simulink model "heli_trim"  (Simulink 7.7)
settings: Solver=FixedStepDiscrete  StartTime=0.0  StopTime=in_N  FixedStep=1  RelTol=1e-3
PostLoadFcn:
  | if exist('helicopter_trim.mat', 'file')
  |     load helicopter_trim.mat;
  | end
undefined symbols (not defined in the file or in its folder): alpha_IERA_IELA_IELA, in_CMD_ini, in_omega_MR, in_omega_TR, in_outside_air_temp, in_pressure_altitude, R_IERA_RA_RA
libraries: UAVdesign_net x2, simulink x2
settings Model: Creator=Emanuel  LastModifiedBy=Emanuel
settings DataIOCC: LimitDataPoints=off  SaveOutput=off  SignalLogging=off
settings OptimizationCC: SimCompilerOptimization=On
settings DebuggingCC: StrictBusMsg=Warning
settings HardwareCC: ProdIntDivRoundTo=Zero  ProdEndianess=LittleEndian  ProdHWDeviceType=Generic->32-bit x86 compatible
settings SFSimCC: SimParseCustomCode=off

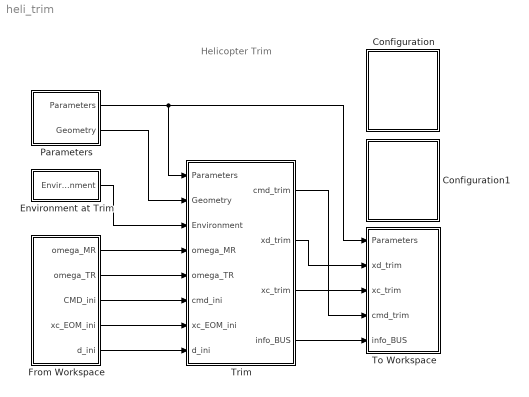
== system heli_trim ==
  note: Helicopter Trim
  Configuration : Subsystem
      settings: OpenFcn=gui_HelicopterTrim;
      mask Display: disp('Double-click\nto configure\nthe\nsimulation')
  Configuration1 : Subsystem
      settings: OpenFcn=graphs_Helicopter_trim;
      mask Display: disp('Double-click\nto display\nthe\ngraphs')
  Environment at Trim : Subsystem
  From Workspace : Subsystem
  Parameters : Subsystem
      mask init:
      | set_param(gcb, 'LinkStatus', 'none');
      settings: OpenFcn=gui_HelicopterParameters( 'Block', [get_param(gcb, 'Parent') '/' get_param(gcb, 'Name')]);
      mask Display:
      | port_label('output', 1, 'Parameters')
      | port_label('output', 2, 'Geometry')
  To Workspace : Subsystem
  Trim : Subsystem  TreatAsAtomicUnit=on
  wires:
  Parameters/2(Geometry) -> Trim/2(Geometry)
  Parameters/1(Parameters) -> Trim/1(Parameters), To Workspace/1(Parameters)
  Trim/2(xd_trim) -> To Workspace/2(xd_trim)
  From Workspace/3(CMD_ini) -> Trim/6(cmd_ini)
  From Workspace/4(xc_EOM_ini) -> Trim/7(xc_EOM_ini)
  From Workspace/5(d_ini) -> Trim/8(d_ini)
  Trim/1(cmd_trim) -> To Workspace/4(cmd_trim)
  Environment at Trim/1(Environment) -> Trim/3(Environment)
  From Workspace/2(omega_TR) -> Trim/5(omega_TR)
  From Workspace/1(omega_MR) -> Trim/4(omega_MR)
  Trim/4(info_BUS) -> To Workspace/5(info_BUS)
  Trim/3(xc_trim) -> To Workspace/3(xc_trim)

== system heli_trim/Configuration ==

== system heli_trim/Configuration1 ==

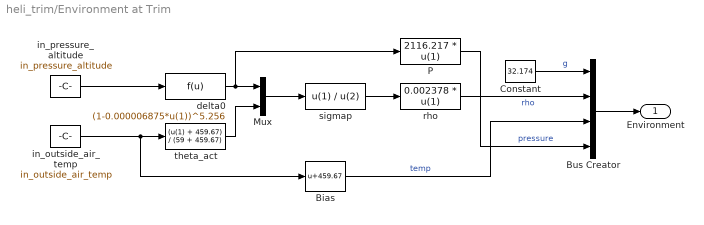
== system heli_trim/Environment at Trim ==
  Bias : Bias  Bias=459.67
  Bus Creator : BusCreator  OutDataTypeStr=Bus: Environment  NonVirtualBus=on
  Constant : Constant  Value=32.174
  Mux : Mux  Inputs=2
  P : Fcn  Expr=2116.217 * u(1)
  delta0 : Fcn  Expr=(1-0.000006875*u(1))^5.256
  in_outside_air_temp : Constant  Value=in_outside_air_temp
  in_pressure_altitude : Constant  Value=in_pressure_altitude
  rho : Fcn  Expr=0.002378 * u(1)
  sigmap : Fcn  Expr=u(1) / u(2)
  theta_act : Fcn  Expr=(u(1) + 459.67) / (59 + 459.67)
  Environment : Outport  OutDataTypeStr=Bus: Environment
  wires:
  sigmap/1 -> rho/1
  theta_act/1 -> Mux/2
  Mux/1 -> sigmap/1
  in_outside_air_temp/1 -> Bias/1, theta_act/1
  delta0/1 -> P/1, Mux/1
  in_pressure_altitude/1 -> delta0/1
  Bus Creator/1 -> Environment/1
  Constant/1 -> Bus Creator/1  "g"
  rho/1 -> Bus Creator/2  "rho"
  Bias/1 -> Bus Creator/3  "temp"
  P/1 -> Bus Creator/4  "pressure"

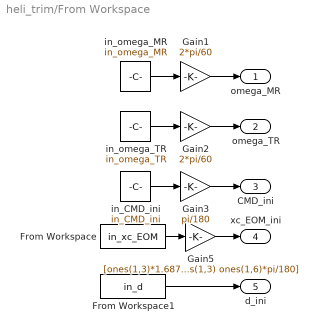
== system heli_trim/From Workspace ==
  From Workspace : FromWorkspace  VariableName=in_xc_EOM  SampleTime=1
  From Workspace1 : FromWorkspace  VariableName=in_d  SampleTime=1
  Gain1 : Gain  Gain=2*pi/60
  Gain2 : Gain  Gain=2*pi/60
  Gain3 : Gain  Gain=pi/180
  Gain5 : Gain  Gain=[ones(1,3)*1.68780986 ones(1,3) ones(1,6)*pi/180]
  in_CMD_ini : Constant  Value=in_CMD_ini
  in_omega_MR : Constant  Value=in_omega_MR
  in_omega_TR : Constant  Value=in_omega_TR
  omega_MR : Outport
  omega_TR : Outport  Port=2
  CMD_ini : Outport  Port=3
  xc_EOM_ini : Outport  Port=4
  d_ini : Outport  Port=5
  wires:
  in_omega_MR/1 -> Gain1/1
  in_omega_TR/1 -> Gain2/1
  in_CMD_ini/1 -> Gain3/1
  From Workspace/1 -> Gain5/1
  Gain1/1 -> omega_MR/1
  Gain2/1 -> omega_TR/1
  Gain3/1 -> CMD_ini/1
  Gain5/1 -> xc_EOM_ini/1
  From Workspace1/1 -> d_ini/1

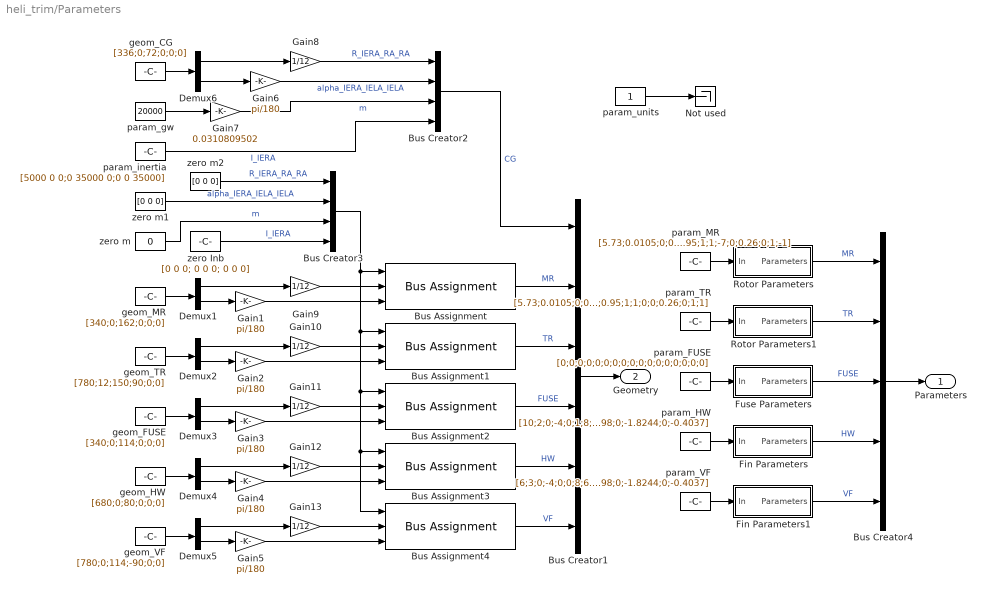
== system heli_trim/Parameters ==
  Bus Assignment{,1..4} (5 alike) : BusAssignment  AssignedSignals=R_IERA_RA_RA,alpha_IERA_IELA_IELA
  Bus Creator1 : BusCreator  Inputs=6
  Bus Creator2 : BusCreator  OutDataTypeStr=Bus: GeometryParameters
  Bus Creator3 : BusCreator  OutDataTypeStr=Bus: GeometryParameters
  Bus Creator4 : BusCreator  Inputs=5
  Demux{1..6} (6 alike) : Demux  Outputs=2
  Fin Parameters : Subsystem
  Fin Parameters1 : Subsystem
  Fuse Parameters : Subsystem
  Gain{1..6} (6 alike) : Gain  Gain=pi/180
  Gain{8..13} (6 alike) : Gain  Gain=1/12
  Gain7 : Gain  Gain=0.0310809502
  Not used : Terminator
  Rotor Parameters : Subsystem
  Rotor Parameters1 : Subsystem
  geom_CG : Constant  Value=[336;0;72;0;0;0]
  geom_FUSE : Constant  Value=[340;0;114;0;0;0]
  geom_HW : Constant  Value=[680;0;80;0;0;0]
  geom_MR : Constant  Value=[340;0;162;0;0;0]
  geom_TR : Constant  Value=[780;12;150;90;0;0]
  geom_VF : Constant  Value=[780;0;114;-90;0;0]
  param_FUSE : Constant  Value=[0;0;0;0;0;0;0;0;0;0;0;0;0;0;0;0;0]
  param_HW : Constant  Value=[10;2;0;-4;0;1;8;6.13;0.9682;1.8898;0;-1.8244;0;-0.4037]
  param_MR : Constant  Value=[5.73;0.0105;0;0.01325;0;-15;0;0;7;30;2.5;0.95;1;1;-7;0;0.26;0;1;-1]
  param_TR : Constant  Value=[5.73;0.0105;0;0.01325;0;-45;0;0;4;6.5;1.25;0.95;1;1;0;0;0.26;0;1;1]
  param_VF : Constant  Value=[6;3;0;-4;0;0;8;6.1311;0.9682;1.8898;0;-1.8244;0;-0.4037]
  param_gw : Constant  Value=20000
  param_inertia : Constant  Value=[5000 0 0;0 35000 0;0 0 35000]
  param_units : Constant
  zero Inb : Constant  Value=[0 0 0; 0 0 0; 0 0 0]
  zero m : Constant  Value=0
  zero m1 : Constant  Value=[0 0 0]
  zero m2 : Constant  Value=[0 0 0]
  Parameters : Outport
  Geometry : Outport  Port=2
  wires:
  Bus Creator2/1 -> Bus Creator1/1  "CG"
  Bus Assignment1/1 -> Bus Creator1/3  "TR"
  Bus Assignment2/1 -> Bus Creator1/4  "FUSE"
  Bus Assignment3/1 -> Bus Creator1/5  "HW"
  Bus Assignment4/1 -> Bus Creator1/6  "VF"
  Bus Creator1/1 -> Geometry/1
  Demux6/1 -> Gain8/1
  Demux6/2 -> Gain6/1
  param_gw/1 -> Gain7/1
  param_inertia/1 -> Bus Creator2/4  "I_IERA"
  Bus Assignment/1 -> Bus Creator1/2  "MR"
  Demux1/1 -> Gain9/1
  Demux1/2 -> Gain1/1
  geom_MR/1 -> Demux1/1
  Demux2/1 -> Gain10/1
  Demux2/2 -> Gain2/1
  geom_TR/1 -> Demux2/1
  Demux3/1 -> Gain11/1
  Demux3/2 -> Gain3/1
  geom_FUSE/1 -> Demux3/1
  Demux4/1 -> Gain12/1
  Demux4/2 -> Gain4/1
  geom_HW/1 -> Demux4/1
  Demux5/1 -> Gain13/1
  Demux5/2 -> Gain5/1
  geom_VF/1 -> Demux5/1
  geom_CG/1 -> Demux6/1
  Bus Creator3/1 -> Bus Assignment/1, Bus Assignment1/1, Bus Assignment2/1, Bus Assignment4/1, Bus Assignment3/1
  zero m/1 -> Bus Creator3/3  "m"
  zero m1/1 -> Bus Creator3/2  "alpha_IERA_IELA_IELA"
  zero Inb/1 -> Bus Creator3/4  "I_IERA"
  zero m2/1 -> Bus Creator3/1  "R_IERA_RA_RA"
  Bus Creator4/1 -> Parameters/1
  Rotor Parameters/1(Parameters) -> Bus Creator4/1  "MR"
  param_MR/1 -> Rotor Parameters/1(In)
  Rotor Parameters1/1(Parameters) -> Bus Creator4/2  "TR"
  param_TR/1 -> Rotor Parameters1/1(In)
  param_FUSE/1 -> Fuse Parameters/1(In)
  Fuse Parameters/1(Parameters) -> Bus Creator4/3  "FUSE"
  param_VF/1 -> Fin Parameters1/1(In)
  Fin Parameters1/1(Parameters) -> Bus Creator4/5  "VF"
  Fin Parameters/1(Parameters) -> Bus Creator4/4  "HW"
  param_HW/1 -> Fin Parameters/1(In)
  Gain1/1 -> Bus Assignment/3
  Gain2/1 -> Bus Assignment1/3
  Gain3/1 -> Bus Assignment2/3
  Gain4/1 -> Bus Assignment3/3
  Gain5/1 -> Bus Assignment4/3
  Gain6/1 -> Bus Creator2/2  "alpha_IERA_IELA_IELA"
  Gain7/1 -> Bus Creator2/3  "m"
  Gain8/1 -> Bus Creator2/1  "R_IERA_RA_RA"
  Gain9/1 -> Bus Assignment/2
  Gain10/1 -> Bus Assignment1/2
  Gain11/1 -> Bus Assignment2/2
  Gain12/1 -> Bus Assignment3/2
  Gain13/1 -> Bus Assignment4/2
  param_units/1 -> Not used/1

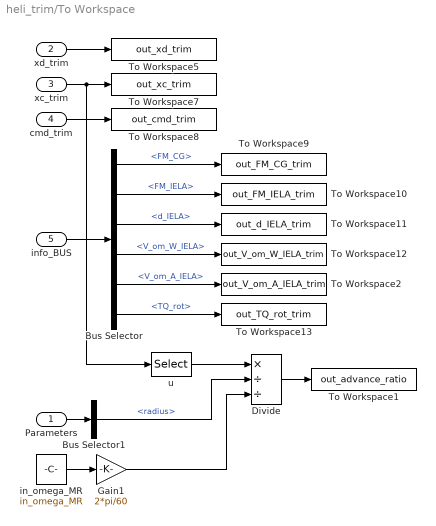
== system heli_trim/To Workspace ==
  Parameters : Inport
  xd_trim : Inport  Port=2
  xc_trim : Inport  Port=3
  cmd_trim : Inport  Port=4
  info_BUS : Inport  Port=5
  Bus Selector : BusSelector  OutputSignals=FM_CG,FM_IELA,d_IELA,V_om_W_IELA,V_om_A_IELA,TQ_rot
  Bus Selector1 : BusSelector  OutputSignals=MR.radius
  Divide : Product  Inputs=*//
  Gain1 : Gain  Gain=2*pi/60
  To Workspace1 : ToWorkspace  VariableName=out_advance_ratio  SampleTime=-1  SaveFormat=Array
  To Workspace10 : ToWorkspace  VariableName=out_FM_IELA_trim  SampleTime=-1  SaveFormat=Array
  To Workspace11 : ToWorkspace  VariableName=out_d_IELA_trim  SampleTime=-1  SaveFormat=Array
  To Workspace12 : ToWorkspace  VariableName=out_V_om_W_IELA_trim  SampleTime=-1  SaveFormat=Array
  To Workspace13 : ToWorkspace  VariableName=out_TQ_rot_trim  SampleTime=-1  SaveFormat=Array
  To Workspace2 : ToWorkspace  VariableName=out_V_om_A_IELA_trim  SampleTime=-1  SaveFormat=Array
  To Workspace5 : ToWorkspace  VariableName=out_xd_trim  SampleTime=-1  SaveFormat=Array
  To Workspace7 : ToWorkspace  VariableName=out_xc_trim  SampleTime=-1  SaveFormat=Array
  To Workspace8 : ToWorkspace  VariableName=out_cmd_trim  SampleTime=-1  SaveFormat=Array
  To Workspace9 : ToWorkspace  VariableName=out_FM_CG_trim  SampleTime=-1  SaveFormat=Array
  in_omega_MR : Constant  Value=in_omega_MR
  u : Selector  InputPortWidth=26  IndexOptions=Index vector (dialog)  Indices=[9]  OutputSizes=1
  wires:
  xd_trim/1 -> To Workspace5/1
  xc_trim/1 -> To Workspace7/1, u/1
  cmd_trim/1 -> To Workspace8/1
  info_BUS/1 -> Bus Selector/1
  Bus Selector/1 -> To Workspace9/1  "<FM_CG>"
  Bus Selector/2 -> To Workspace10/1  "<FM_IELA>"
  Bus Selector/3 -> To Workspace11/1  "<d_IELA>"
  Bus Selector/4 -> To Workspace12/1  "<V_om_W_IELA>"
  Bus Selector/6 -> To Workspace13/1  "<TQ_rot>"
  Parameters/1 -> Bus Selector1/1
  in_omega_MR/1 -> Gain1/1
  Bus Selector1/1 -> Divide/2  "<radius>"
  Gain1/1 -> Divide/3
  u/1 -> Divide/1
  Divide/1 -> To Workspace1/1
  Bus Selector/5 -> To Workspace2/1  "<V_om_A_IELA>"

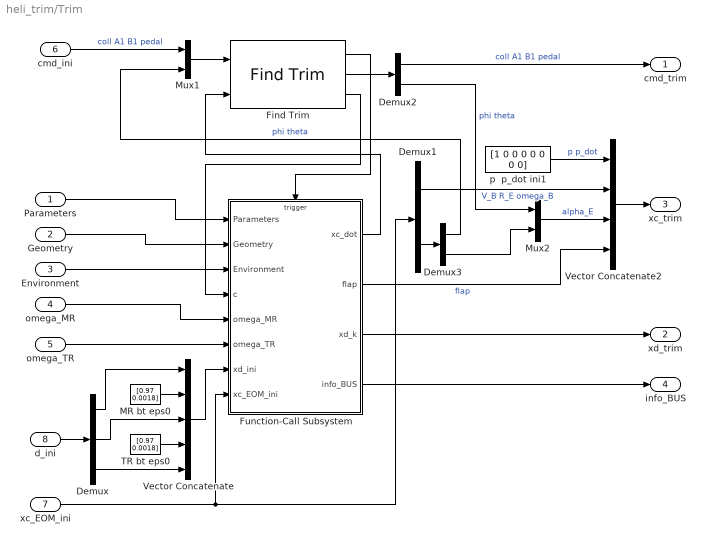
== system heli_trim/Trim ==
  Parameters : Inport
  Geometry : Inport  Port=2
  Environment : Inport  Port=3
  omega_MR : Inport  Port=4
  omega_TR : Inport  Port=5
  cmd_ini : Inport  Port=6
  xc_EOM_ini : Inport  Port=7
  d_ini : Inport  Port=8
  Demux : Demux  Outputs=[3 3 9]
  Demux1 : Demux  Outputs=[9 3]
  Demux2 : Demux  Outputs=[4 2]
  Demux3 : Demux  Outputs=[2 1]
  Find Trim : UAVdesign_net/Utilities/Numeric Perturbation/Find Trim  NumFInputs=6  NumFOutputs=6  RunOnce=off  SampleTime=-1
  Function-Call Subsystem : Subsystem  TreatAsAtomicUnit=on
  MR bt eps0 : Constant  Value=[0.97 0.0018]
  Mux1 : Mux  Inputs=2
  Mux2 : Mux  Inputs=2
  TR bt eps0 : Constant  Value=[0.97 0.0018]
  Vector Concatenate : Concatenate  NumInputs=5  Mode=Vector
  Vector Concatenate2 : Concatenate  NumInputs=4  Mode=Vector
  p  p_dot ini1 : Constant  Value="[1 0 0 0  0 0 0 0]"
  cmd_trim : Outport
  xd_trim : Outport  Port=2
  xc_trim : Outport  Port=3
  info_BUS : Outport  Port=4
  wires:
  Geometry/1 -> Function-Call Subsystem/2(Geometry)
  Parameters/1 -> Function-Call Subsystem/1(Parameters)
  omega_MR/1 -> Function-Call Subsystem/5(omega_MR)
  xc_EOM_ini/1 -> Function-Call Subsystem/8(xc_EOM_ini), Demux1/1
  omega_TR/1 -> Function-Call Subsystem/6(omega_TR)
  Find Trim/3 -> Function-Call Subsystem/4(c)
  Function-Call Subsystem/1(xc_dot) -> Find Trim/2
  Find Trim/1 -> Function-Call Subsystem/Trigger
  Function-Call Subsystem/3(xd_k) -> xd_trim/1
  d_ini/1 -> Demux/1
  Demux/1 -> Vector Concatenate/1
  MR bt eps0/1 -> Vector Concatenate/2
  Demux/2 -> Vector Concatenate/3
  TR bt eps0/1 -> Vector Concatenate/4
  Demux/3 -> Vector Concatenate/5
  Vector Concatenate/1 -> Function-Call Subsystem/7(xd_ini)
  Find Trim/2 -> Demux2/1
  Demux2/1 -> cmd_trim/1  "coll A1 B1 pedal"
  Mux1/1 -> Find Trim/1
  cmd_ini/1 -> Mux1/1  "coll A1 B1 pedal"
  Vector Concatenate2/1 -> xc_trim/1
  p  p_dot ini1/1 -> Vector Concatenate2/1  "p p_dot"
  Demux1/1 -> Vector Concatenate2/2  "V_B R_E omega_B"
  Mux2/1 -> Vector Concatenate2/3  "alpha_E"
  Function-Call Subsystem/2(flap) -> Vector Concatenate2/4  "flap"
  Demux3/2 -> Mux2/2
  Demux1/2 -> Demux3/1
  Demux2/2 -> Mux2/1  "phi theta"
  Demux3/1 -> Mux1/2  "phi theta"
  Environment/1 -> Function-Call Subsystem/3(Environment)
  Function-Call Subsystem/4(info_BUS) -> info_BUS/1

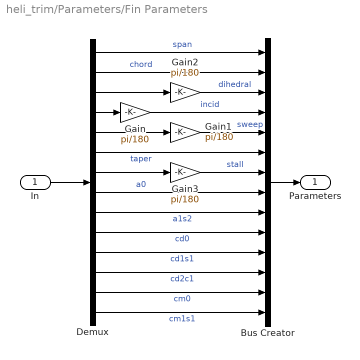
== system heli_trim/Parameters/Fin Parameters ==
  In : Inport
  Bus Creator : BusCreator  Inputs=14  OutDataTypeStr=Bus: FinParameters  NonVirtualBus=on
  Demux : Demux  Outputs=14
  Gain{,1..3} (4 alike) : Gain  Gain=pi/180
  Parameters : Outport  OutDataTypeStr=Bus: FinParameters
  wires:
  In/1 -> Demux/1
  Bus Creator/1 -> Parameters/1
  Demux/1 -> Bus Creator/1  "span"
  Demux/2 -> Bus Creator/2  "chord"
  Demux/3 -> Gain2/1
  Gain2/1 -> Bus Creator/3  "dihedral"
  Demux/4 -> Gain/1
  Gain/1 -> Bus Creator/4  "incid"
  Gain1/1 -> Bus Creator/5  "sweep"
  Demux/5 -> Gain1/1
  Demux/6 -> Bus Creator/6  "taper"
  Demux/7 -> Gain3/1
  Gain3/1 -> Bus Creator/7  "stall"
  Demux/8 -> Bus Creator/8  "a0"
  Demux/9 -> Bus Creator/9  "a1s2"
  Demux/10 -> Bus Creator/10  "cd0"
  Demux/11 -> Bus Creator/11  "cd1s1"
  Demux/12 -> Bus Creator/12  "cd2c1"
  Demux/13 -> Bus Creator/13  "cm0"
  Demux/14 -> Bus Creator/14  "cm1s1"

== system heli_trim/Parameters/Fin Parameters1 ==
  In : Inport
  Bus Creator : BusCreator  Inputs=14  OutDataTypeStr=Bus: FinParameters  NonVirtualBus=on
  Demux : Demux  Outputs=14
  Gain{,1..3} (4 alike) : Gain  Gain=pi/180
  Parameters : Outport  OutDataTypeStr=Bus: FinParameters
  wires:
  Demux/14 -> Bus Creator/14  "cm1s1"
  Demux/13 -> Bus Creator/13  "cm0"
  Demux/12 -> Bus Creator/12  "cd2c1"
  Demux/11 -> Bus Creator/11  "cd1s1"
  Demux/10 -> Bus Creator/10  "cd0"
  Demux/9 -> Bus Creator/9  "a1s2"
  Demux/8 -> Bus Creator/8  "a0"
  Gain3/1 -> Bus Creator/7  "stall"
  Demux/7 -> Gain3/1
  Demux/6 -> Bus Creator/6  "taper"
  Demux/5 -> Gain1/1
  Gain1/1 -> Bus Creator/5  "sweep"
  Gain/1 -> Bus Creator/4  "incid"
  Demux/4 -> Gain/1
  Gain2/1 -> Bus Creator/3  "dihedral"
  Demux/3 -> Gain2/1
  Demux/2 -> Bus Creator/2  "chord"
  Demux/1 -> Bus Creator/1  "span"
  Bus Creator/1 -> Parameters/1
  In/1 -> Demux/1

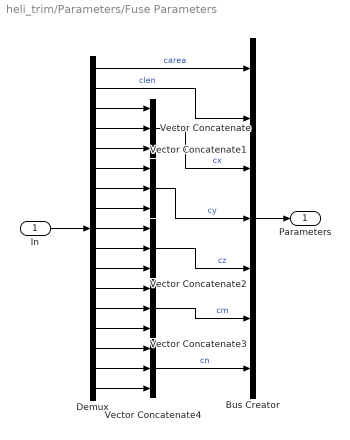
== system heli_trim/Parameters/Fuse Parameters ==
  In : Inport
  Bus Creator : BusCreator  Inputs=7  OutDataTypeStr=Bus: FuselageParameters  NonVirtualBus=on
  Demux : Demux  Outputs=17
  Vector Concatenate{,1..4} (5 alike) : Concatenate  NumInputs=3  Mode=Vector
  Parameters : Outport  OutDataTypeStr=Bus: FuselageParameters
  wires:
  Demux/1 -> Bus Creator/1  "carea"
  Bus Creator/1 -> Parameters/1
  In/1 -> Demux/1
  Demux/2 -> Bus Creator/2  "clen"
  Demux/3 -> Vector Concatenate/1
  Demux/4 -> Vector Concatenate/2
  Demux/5 -> Vector Concatenate/3
  Vector Concatenate/1 -> Bus Creator/3  "cx"
  Demux/6 -> Vector Concatenate1/1
  Demux/7 -> Vector Concatenate1/2
  Demux/8 -> Vector Concatenate1/3
  Vector Concatenate1/1 -> Bus Creator/4  "cy"
  Demux/9 -> Vector Concatenate2/1
  Demux/10 -> Vector Concatenate2/2
  Demux/11 -> Vector Concatenate2/3
  Vector Concatenate2/1 -> Bus Creator/5  "cz"
  Demux/12 -> Vector Concatenate3/1
  Demux/13 -> Vector Concatenate3/2
  Demux/14 -> Vector Concatenate3/3
  Demux/15 -> Vector Concatenate4/1
  Demux/16 -> Vector Concatenate4/2
  Demux/17 -> Vector Concatenate4/3
  Vector Concatenate3/1 -> Bus Creator/6  "cm"
  Vector Concatenate4/1 -> Bus Creator/7  "cn"

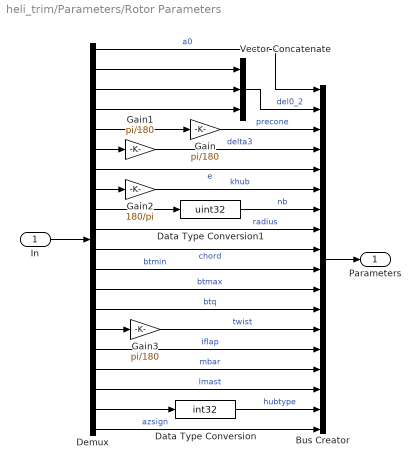
== system heli_trim/Parameters/Rotor Parameters ==
  In : Inport
  Bus Creator : BusCreator  Inputs=18  OutDataTypeStr=Bus: RotorParameters  NonVirtualBus=on
  Data Type Conversion : DataTypeConversion  OutDataTypeStr=int32  RndMeth=Nearest
  Data Type Conversion1 : DataTypeConversion  OutDataTypeStr=uint32  RndMeth=Nearest
  Demux : Demux  Outputs=20
  Gain : Gain  Gain=pi/180
  Gain1 : Gain  Gain=pi/180
  Gain2 : Gain  Gain=180/pi
  Gain3 : Gain  Gain=pi/180
  Vector Concatenate : Concatenate  NumInputs=3  Mode=Vector
  Parameters : Outport  OutDataTypeStr=Bus: RotorParameters
  wires:
  Demux/20 -> Bus Creator/18  "azsign"
  Demux/18 -> Bus Creator/16  "lmast"
  Demux/17 -> Bus Creator/15  "mbar"
  Demux/16 -> Bus Creator/14  "iflap"
  Demux/13 -> Bus Creator/11  "btmax"
  Demux/1 -> Bus Creator/1  "a0"
  Bus Creator/1 -> Parameters/1
  Demux/4 -> Vector Concatenate/3
  Demux/3 -> Vector Concatenate/2
  Demux/2 -> Vector Concatenate/1
  Vector Concatenate/1 -> Bus Creator/2  "del0_2"
  In/1 -> Demux/1
  Data Type Conversion/1 -> Bus Creator/17  "hubtype"
  Demux/19 -> Data Type Conversion/1
  Gain/1 -> Bus Creator/3  "precone"
  Gain1/1 -> Bus Creator/4  "delta3"
  Gain2/1 -> Bus Creator/6  "khub"
  Gain3/1 -> Bus Creator/13  "twist"
  Demux/5 -> Gain/1
  Demux/6 -> Gain1/1
  Demux/7 -> Bus Creator/5  "e"
  Demux/8 -> Gain2/1
  Data Type Conversion1/1 -> Bus Creator/7  "nb"
  Demux/9 -> Data Type Conversion1/1
  Demux/10 -> Bus Creator/8  "radius"
  Demux/11 -> Bus Creator/9  "chord"
  Demux/12 -> Bus Creator/10  "btmin"
  Demux/15 -> Gain3/1
  Demux/14 -> Bus Creator/12  "btq"

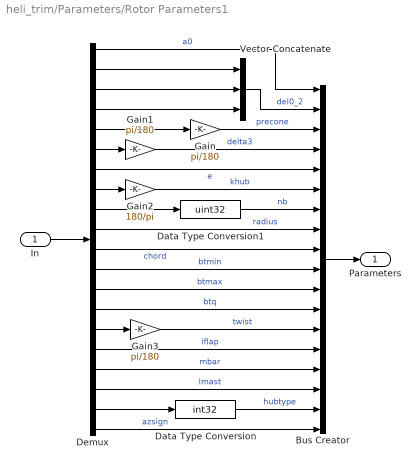
== system heli_trim/Parameters/Rotor Parameters1 ==
  In : Inport
  Bus Creator : BusCreator  Inputs=18  OutDataTypeStr=Bus: RotorParameters  NonVirtualBus=on
  Data Type Conversion : DataTypeConversion  OutDataTypeStr=int32  RndMeth=Nearest
  Data Type Conversion1 : DataTypeConversion  OutDataTypeStr=uint32  RndMeth=Nearest
  Demux : Demux  Outputs=20
  Gain : Gain  Gain=pi/180
  Gain1 : Gain  Gain=pi/180
  Gain2 : Gain  Gain=180/pi
  Gain3 : Gain  Gain=pi/180
  Vector Concatenate : Concatenate  NumInputs=3  Mode=Vector
  Parameters : Outport  OutDataTypeStr=Bus: RotorParameters
  wires:
  Demux/14 -> Bus Creator/12  "btq"
  Demux/15 -> Gain3/1
  Demux/12 -> Bus Creator/10  "btmin"
  Demux/11 -> Bus Creator/9  "chord"
  Demux/10 -> Bus Creator/8  "radius"
  Demux/9 -> Data Type Conversion1/1
  Data Type Conversion1/1 -> Bus Creator/7  "nb"
  Demux/8 -> Gain2/1
  Demux/7 -> Bus Creator/5  "e"
  Demux/6 -> Gain1/1
  Demux/5 -> Gain/1
  Gain3/1 -> Bus Creator/13  "twist"
  Gain2/1 -> Bus Creator/6  "khub"
  Gain1/1 -> Bus Creator/4  "delta3"
  Gain/1 -> Bus Creator/3  "precone"
  Demux/19 -> Data Type Conversion/1
  Data Type Conversion/1 -> Bus Creator/17  "hubtype"
  In/1 -> Demux/1
  Vector Concatenate/1 -> Bus Creator/2  "del0_2"
  Demux/2 -> Vector Concatenate/1
  Demux/3 -> Vector Concatenate/2
  Demux/4 -> Vector Concatenate/3
  Bus Creator/1 -> Parameters/1
  Demux/1 -> Bus Creator/1  "a0"
  Demux/13 -> Bus Creator/11  "btmax"
  Demux/16 -> Bus Creator/14  "iflap"
  Demux/17 -> Bus Creator/15  "mbar"
  Demux/18 -> Bus Creator/16  "lmast"
  Demux/20 -> Bus Creator/18  "azsign"

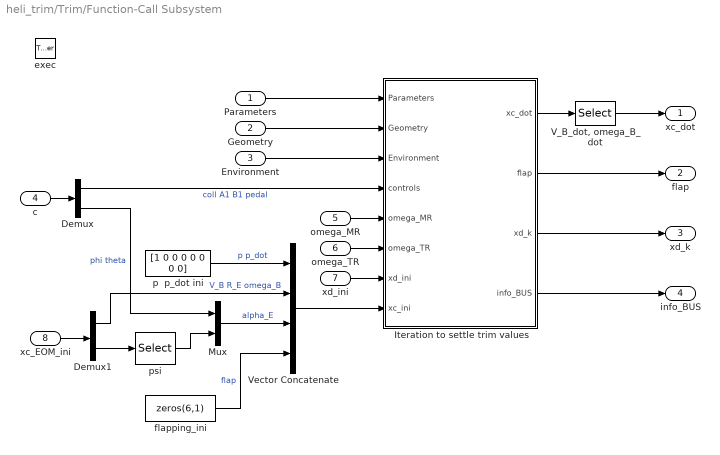
== system heli_trim/Trim/Function-Call Subsystem ==
  Parameters : Inport
  Geometry : Inport  Port=2
  Environment : Inport  Port=3
  c : Inport  Port=4
  omega_MR : Inport  Port=5
  omega_TR : Inport  Port=6
  xd_ini : Inport  Port=7
  xc_EOM_ini : Inport  Port=8
  exec : TriggerPort  TriggerType=function-call
  Demux : Demux  Outputs=[4 2]
  Demux1 : Demux  Outputs=[9 3]
  Iteration to settle trim values : Subsystem  TreatAsAtomicUnit=on
  Mux : Mux  Inputs=2
  "V_B_dot, omega_B_dot" : Selector  InputPortWidth=26  IndexOptions=Index vector (dialog)  Indices=[9:11 15:17]  OutputSizes=1
  Vector Concatenate : Concatenate  NumInputs=4  Mode=Vector
  flapping_ini : Constant  Value=zeros(6,1)
  p  p_dot ini : Constant  Value="[1 0 0 0  0 0 0 0]"
  psi : Selector  InputPortWidth=3  IndexOptions=Index vector (dialog)  Indices=[3]  OutputSizes=1
  xc_dot : Outport
  flap : Outport  Port=2
  xd_k : Outport  Port=3
  info_BUS : Outport  Port=4
  wires:
  Parameters/1 -> Iteration to settle trim values/1(Parameters)
  Geometry/1 -> Iteration to settle trim values/2(Geometry)
  omega_MR/1 -> Iteration to settle trim values/5(omega_MR)
  omega_TR/1 -> Iteration to settle trim values/6(omega_TR)
  c/1 -> Demux/1
  Demux/1 -> Iteration to settle trim values/4(controls)  "coll A1 B1 pedal"
  xd_ini/1 -> Iteration to settle trim values/7(xd_ini)
  Vector Concatenate/1 -> Iteration to settle trim values/8(xc_ini)
  p  p_dot ini/1 -> Vector Concatenate/1  "p p_dot"
  xc_EOM_ini/1 -> Demux1/1
  Demux1/1 -> Vector Concatenate/2  "V_B R_E omega_B"
  Mux/1 -> Vector Concatenate/3  "alpha_E"
  Demux/2 -> Mux/1  "phi theta"
  flapping_ini/1 -> Vector Concatenate/4  "flap"
  Iteration to settle trim values/1(xc_dot) -> "V_B_dot, omega_B_dot"/1
  "V_B_dot, omega_B_dot"/1 -> xc_dot/1
  Iteration to settle trim values/2(flap) -> flap/1
  Iteration to settle trim values/3(xd_k) -> xd_k/1
  psi/1 -> Mux/2
  Demux1/2 -> psi/1
  Environment/1 -> Iteration to settle trim values/3(Environment)
  Iteration to settle trim values/4(info_BUS) -> info_BUS/1

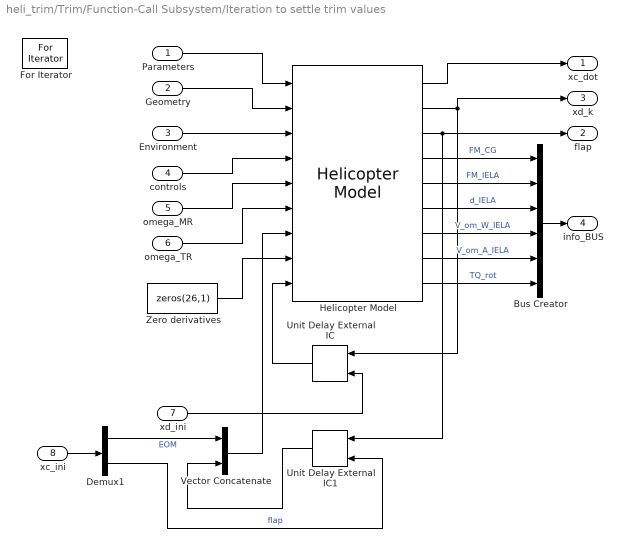
== system heli_trim/Trim/Function-Call Subsystem/Iteration to settle trim values ==
  Parameters : Inport
  Geometry : Inport  Port=2
  Environment : Inport  Port=3
  controls : Inport  Port=4
  omega_MR : Inport  Port=5
  omega_TR : Inport  Port=6
  xd_ini : Inport  Port=7
  xc_ini : Inport  Port=8
  Bus Creator : BusCreator  Inputs=6
  Demux1 : Demux  Outputs=[20 6]
  For Iterator : ForIterator  ResetStates=reset  IterationLimit=20  ShowIterationPort=off
  Helicopter Model : UAVdesign_net/Vehicle Models/Helicopter Model  SystemSampleTime=-1
  Unit Delay External IC : simulink/Additional Math & Discrete/Additional Discrete/Unit Delay External IC  SystemSampleTime=-1  tsamp=-1
  Unit Delay External IC1 : simulink/Additional Math & Discrete/Additional Discrete/Unit Delay External IC  SystemSampleTime=-1  tsamp=-1
  Vector Concatenate : Concatenate  Mode=Vector
  Zero derivatives : Constant  Value=zeros(26,1)
  xc_dot : Outport
  flap : Outport  Port=2
  xd_k : Outport  Port=3
  info_BUS : Outport  Port=4
  wires:
  Unit Delay External IC1/1 -> Vector Concatenate/2
  Demux1/2 -> Unit Delay External IC1/2  "flap"
  Demux1/1 -> Vector Concatenate/1  "EOM"
  Vector Concatenate/1 -> Helicopter Model/7
  xc_ini/1 -> Demux1/1
  Helicopter Model/3 -> Unit Delay External IC1/1, flap/1
  Zero derivatives/1 -> Helicopter Model/8
  xd_ini/1 -> Unit Delay External IC/2
  omega_TR/1 -> Helicopter Model/6
  omega_MR/1 -> Helicopter Model/5
  controls/1 -> Helicopter Model/4
  Environment/1 -> Helicopter Model/3
  Geometry/1 -> Helicopter Model/2
  Parameters/1 -> Helicopter Model/1
  Helicopter Model/1 -> xc_dot/1
  Helicopter Model/2 -> Unit Delay External IC/1, xd_k/1
  Unit Delay External IC/1 -> Helicopter Model/9
  Bus Creator/1 -> info_BUS/1
  Helicopter Model/4 -> Bus Creator/1  "FM_CG"
  Helicopter Model/5 -> Bus Creator/2  "FM_IELA"
  Helicopter Model/6 -> Bus Creator/3  "d_IELA"
  Helicopter Model/7 -> Bus Creator/4  "V_om_W_IELA"
  Helicopter Model/8 -> Bus Creator/5  "V_om_A_IELA"
  Helicopter Model/9 -> Bus Creator/6  "TQ_rot"
